simulink model "controle_com_portas"  (R2015a)
settings: Solver=ode45  StartTime=0.0  StopTime=2000  RelTol=1e-4
settings Model: Creator=pedro  LastModifiedBy=Administrator
settings OptimizationCC: ExpressionDepthLimit=2147483647
settings DebuggingCC: SolverPrmCheckMsg=warning  StateNameClashWarn=warning

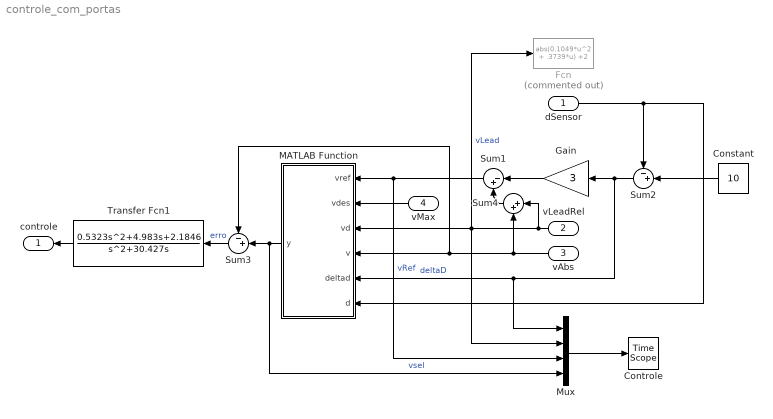
== system controle_com_portas ==
  dSensor : Inport
  vLeadRel : Inport  Port=2
  vAbs : Inport  Port=3
  vMax : Inport  Port=4
  Constant : Constant  Value=10
  Controle : TimeScope
  Fcn : Fcn  Commented=on  Expr=abs(0.1049*u^2 + .3739*u) +2
  Gain : Gain  Gain=3
  MATLAB Function : MATLAB Function  TreatAsAtomicUnit=on
  Mux : Mux
  Sum1 : Sum  Inputs=|-+
  Sum2 : Sum  Inputs=-+|
  Sum3 : Sum  Inputs=-+|
  Sum4 : Sum  Inputs=|++
  Transfer Fcn1 : TransferFcn  Numerator=[0.5323 4.983 2.1846]  Denominator=[1 30.427 0]
  controle : Outport
  wires:
  dSensor/1 -> MATLAB Function/6(d), Sum2/1
  Sum2/1 -> Gain/1, Mux/1, MATLAB Function/5(deltad)  "deltaD"
  Gain/1 -> Sum1/1
  MATLAB Function/1(y) -> Sum3/2, Mux/4  "vsel"
  Sum1/1 -> Mux/3, MATLAB Function/1(vref)  "vRef"
  vMax/1 -> MATLAB Function/2(vdes)
  Sum3/1 -> Transfer Fcn1/1  "erro"
  Transfer Fcn1/1 -> controle/1
  vAbs/1 -> Sum4/2, MATLAB Function/4(v), Sum3/1
  vLeadRel/1 -> Sum4/1, Mux/2, MATLAB Function/3(vd), Fcn/1  "vLead"
  Sum4/1 -> Sum1/2
  Mux/1 -> Controle/1
  Constant/1 -> Sum2/2

== matlab function controle_com_portas/MATLAB Function ==
  data: vref input; vdes input; y output; vd input; v input; deltad input; d input
function y   = fcn(vref, vdes, vd, v, deltad,d)
%#codegen
%if(deltad<0)
%    y=vdes;
%end

%if(deltad>0 && v<vref)
%    y=vref;
%end


% if(deltad<0)
%     y=vdes;
% elseif(v<vref)
%     y=min(vdes, vref);
% elseif(vd<0)
%     y=min(vdes, vref);
% else
%     y=vdes;
% end

%if(d >=10)

    if(deltad<0)
        y=vdes;
    else
        if(v<vref)
            y=min(vdes, vref);
        else
            if(vd < 0)
                y=min(vdes, vref);
            else
                y = vdes;
            end
        end
    end
% else
%     y = 0;
%     flag = 0;
%end
